simulink model "EvBoltCalib_Lat_v1_comb_GBSRoto"  (R2022b)
settings: configuration reference "ConfigSetDesktopFixedStep" (kept outside this file)
PreLoadFcn:
  | VSS_BICYCLE=Simulink.Variant('Dual=0');
  | VSS_DUAL=Simulink.Variant('Dual=1');
  | Dual=1;
model workspace (MAT data in the model file):
  Gas = 0.383333333333
undefined symbols (not defined in the file or in its folder): AccelCmd, ActTqLF_Nm_, ActTqLR_Nm_, ActTqRF_Nm_, ActTqRR_Nm_, BattChargeLimitMaxPwr, BattChargeLimitSocBpts, BattChargeLimitTbl, BattChrgCapcty, BattDischargeLimitSocBpts, BattDischargeLimitTbl, BattDischargeMaxPwr, BattNumCellsParallel, BattNumCellsSeries, BattOpenVoltCapBpts, BattOpenVoltTbl, BattResistSocBpts, BattResistTbl, BattResistTempBpts, BrakeMaxPrs, BrakeMaxTrq, ChassisDistCg2FrontAxle, ChassisDistCg2RearAxle, ChassisVehMass, CltchCmd, DecelCmd, DiffRatio, DiscIntNeverNeededParam, EnvGravCnst, EnvPrs, EnvTemp, FuelSpecificGrav, GearCmd, h, InitStates, lgSw, MtrEffSpdBpts, MtrEffTbl, MtrEffTrqBpts, MtrPwrMax, MtrTrqMax, SteeringCmd, SupvsryCtrlRegenBrkCutOffTbl, SupvsryCtrlRegenSpdBpts, TestScnrioCycleNum, VEH
libraries: VSIGenLib x39, simulink x25, etargetslib x24, vehdynlibtire x8, vehdynlibsuspension x7, vehdynlibtirecommon x7, autolibutils x5, autolibshared x5, CarMaker4SL x4, VsrLibWheel x4, sharedtransform x3, slrealtimeiplib x3
(part 11 of 11)

== system EvBoltCalib_Lat_v1_comb_GBSRoto/Subsystem/Vehicle/Vehicle Dynamics/Vehicle 14DOF/Wheels and Tires/VDBS/Tires/MF Tires/kappa ==
  In1 : Inport
  In2 : Inport  Port=2
  In3 : Inport  Port=3
  In4 : Inport  Port=4
  Bus Selector{,1..3} (4 alike) : BusSelector  OutputSignals=Kappa
  Vector Concatenate : Concatenate  NumInputs=4
  Out1 : Outport  VectorParamsAs1DForOutWhenUnconnected=off
  wires:
  Bus Selector3/1 -> Vector Concatenate/4  "<Kappa>"
  Bus Selector2/1 -> Vector Concatenate/3  "<Kappa>"
  Bus Selector1/1 -> Vector Concatenate/2  "<Kappa>"
  In4/1 -> Bus Selector3/1
  In3/1 -> Bus Selector2/1
  In2/1 -> Bus Selector1/1
  Bus Selector/1 -> Vector Concatenate/1  "<Kappa>"
  In1/1 -> Bus Selector/1
  Vector Concatenate/1 -> Out1/1

== system EvBoltCalib_Lat_v1_comb_GBSRoto/Subsystem/Vehicle/Vehicle Dynamics/Vehicle 14DOF/Wheels and Tires/VDBS/Tires/MF Tires/omega ==
  In1 : Inport
  In2 : Inport  Port=2
  In3 : Inport  Port=3
  In4 : Inport  Port=4
  Bus Selector{,1..3} (4 alike) : BusSelector  OutputSignals=Omega
  Vector Concatenate : Concatenate  NumInputs=4
  Out1 : Outport  VectorParamsAs1DForOutWhenUnconnected=off
  wires:
  In1/1 -> Bus Selector/1
  Bus Selector/1 -> Vector Concatenate/1  "<Omega>"
  In2/1 -> Bus Selector1/1
  In3/1 -> Bus Selector2/1
  In4/1 -> Bus Selector3/1
  Bus Selector1/1 -> Vector Concatenate/2  "<Omega>"
  Bus Selector2/1 -> Vector Concatenate/3  "<Omega>"
  Bus Selector3/1 -> Vector Concatenate/4  "<Omega>"
  Vector Concatenate/1 -> Out1/1

== system EvBoltCalib_Lat_v1_comb_GBSRoto/Subsystem/Vehicle/Vehicle Dynamics/Vehicle 14DOF/Wheels and Tires/VDBS/Tires/MF Tires/z ==
  In1 : Inport
  In2 : Inport  Port=2
  In3 : Inport  Port=3
  In4 : Inport  Port=4
  Bus Selector{,1..3} (4 alike) : BusSelector  OutputSignals=z
  Vector Concatenate : Concatenate  NumInputs=4
  Out1 : Outport  VectorParamsAs1DForOutWhenUnconnected=off
  wires:
  Bus Selector3/1 -> Vector Concatenate/4  "<z>"
  Bus Selector2/1 -> Vector Concatenate/3  "<z>"
  Bus Selector1/1 -> Vector Concatenate/2  "<z>"
  In4/1 -> Bus Selector3/1
  In3/1 -> Bus Selector2/1
  In2/1 -> Bus Selector1/1
  Bus Selector/1 -> Vector Concatenate/1  "<z>"
  In1/1 -> Bus Selector/1
  Vector Concatenate/1 -> Out1/1

== system EvBoltCalib_Lat_v1_comb_GBSRoto/Subsystem/Vehicle/Vehicle Dynamics/Vehicle 14DOF/Wheels and Tires/VDBS/Tires/MF Tires/zdot ==
  In1 : Inport
  In2 : Inport  Port=2
  In3 : Inport  Port=3
  In4 : Inport  Port=4
  Bus Selector{,1..3} (4 alike) : BusSelector  OutputSignals=zdot
  Vector Concatenate : Concatenate  NumInputs=4
  Out1 : Outport  VectorParamsAs1DForOutWhenUnconnected=off
  wires:
  Vector Concatenate/1 -> Out1/1
  In1/1 -> Bus Selector/1
  Bus Selector/1 -> Vector Concatenate/1  "<zdot>"
  In2/1 -> Bus Selector1/1
  In3/1 -> Bus Selector2/1
  In4/1 -> Bus Selector3/1
  Bus Selector1/1 -> Vector Concatenate/2  "<zdot>"
  Bus Selector2/1 -> Vector Concatenate/3  "<zdot>"
  Bus Selector3/1 -> Vector Concatenate/4  "<zdot>"

== matlab function EvBoltCalib_Lat_v1_comb_GBSRoto/Subsystem/Vehicle/Vehicle Dynamics/Vehicle 14DOF/Rototest and ORNL Interface/To Rototest with Band-Aid/RotoTestEthTx/MATLAB Function ==
  data: SpTqRR input; y output; SpTqLR input; SpTqRF input; SpTqLF input; SystemActive input
function y = fcn(SpTqRR, SpTqLR, SpTqRF, SpTqLF, SystemActive)

y = 0;
if SpTqRR == 1 && SystemActive == 0
    y = 30;
elseif SpTqRR == 0 && SystemActive == 0
    y = 0;
elseif SpTqRR == 1 && SystemActive == 1
    y = 31;
elseif SpTqRR == 0 && SystemActive == 1
    y = 1;
end

y = uint8(y);

== matlab function EvBoltCalib_Lat_v1_comb_GBSRoto/Subsystem/Vehicle/Vehicle Dynamics/Vehicle 7DOF/For 3D Visualization ==
  data: angles output size=3; angleIn input size=3; GeomXYZ output size=3; GemoXYZIn input size=3; GroundZ input size=4; trackW parameter; wheelB parameter
function [angles,GeomXYZ]= three26(angleIn, GemoXYZIn, GroundZ,trackW, wheelB)%#codegen
coder.allowpcode('plain')
% Copyright 2018 The MathWorks, Inc.
[angles,GeomXYZ]= vdynthree2six(angleIn, GemoXYZIn, GroundZ,trackW, wheelB);

== matlab function EvBoltCalib_Lat_v1_comb_GBSRoto/Subsystem/Vehicle/Vehicle Dynamics/Vehicle 14DOF/Rototest and ORNL Interface/Get Wheel Spd Cmd Based on Wheel Dynamics/Whl Dynamics & Format CM Powertrain Signal/Subsystem/MATLAB Function ==
  data: axleTorq input; switchFlag output; wheelSpd input
function switchFlag = fcn(axleTorq, wheelSpd)

% if braking and vehicle has stopped
if (abs(axleTorq) < 1e-5 && abs(wheelSpd) < 1e-5)
    switchFlag = 1;
else
    switchFlag = 0;
end

== matlab function EvBoltCalib_Lat_v1_comb_GBSRoto/Subsystem/Vehicle/Vehicle Dynamics/Vehicle 14DOF/Rototest and ORNL Interface/Get Wheel Spd Cmd Based on Wheel Dynamics/Whl Dynamics & Format CM Powertrain Signal/Subsystem2/MATLAB Function ==
  data: axleTorq input; switchFlag output; wheelSpd input
function switchFlag = fcn(axleTorq, wheelSpd)

% if braking and vehicle has stopped
if (abs(axleTorq) < 1e-5 && abs(wheelSpd) < 1e-5)
    switchFlag = 1;
else
    switchFlag = 0;
end

== matlab function EvBoltCalib_Lat_v1_comb_GBSRoto/Subsystem/Vehicle/Vehicle Dynamics/Vehicle 14DOF/Rototest and ORNL Interface/Get Wheel Spd Cmd Based on Wheel Dynamics/Whl Dynamics & Format CM Powertrain Signal/Subsystem3/MATLAB Function ==
  data: axleTorq input; switchFlag output; wheelSpd input
function switchFlag = fcn(axleTorq, wheelSpd)

% if braking and vehicle has stopped
if (abs(axleTorq) < 1e-5 && abs(wheelSpd) < 1e-5)
    switchFlag = 1;
else
    switchFlag = 0;
end

== matlab function EvBoltCalib_Lat_v1_comb_GBSRoto/Subsystem/Vehicle/Vehicle Dynamics/Vehicle 14DOF/Rototest and ORNL Interface/Get Wheel Spd Cmd Based on Wheel Dynamics/Whl Dynamics & Format CM Powertrain Signal/Subsystem4/MATLAB Function ==
  data: axleTorq input; switchFlag output; wheelSpd input
function switchFlag = fcn(axleTorq, wheelSpd)

% if braking and vehicle has stopped
if (abs(axleTorq) < 1e-5 && abs(wheelSpd) < 1e-5)
    switchFlag = 1;
else
    switchFlag = 0;
end

== stateflow chart EvBoltCalib_Lat_v1_comb_GBSRoto/Subsystem/Vehicle/Vehicle Dynamics/Vehicle 14DOF/Rototest and ORNL Interface/To Rototest with Band-Aid/Band-Aid/Band-Aid ==
  state dStop
    en:
    OutMode = 0;
    State = 3;
  state Running
    state SpeedMode
      en:
      OutMode = 1;
      state Blend
        en:
        OutSpd = InSpd;
        State = 0.1;
      state Driving
        du:
        OutSpd = InSpd;
        State = 0.2;
      (default) -> Blend
      Blend -> Driving
    state TorqueMode
      en:
      OutMode = 0;
      du:
      State = 1;
    (default) -> SpeedMode
    TorqueMode -> Blend : [after(SettleTime, sec) || ...
        | ~BrkSw]
    SpeedMode -> TorqueMode : [(any(InSpd < SpdLatchThr) && ...
        | (VehSpd_kph < VehSpdThr_kph) && BrkSw)]
  note: The vehicle will enter speed mode (driving) if:
      | The vehicle has been in torque mode for a calibrated time (settleTime) AND
      | The Input Speed (InSpd) is greater than a Launch Treshold (LaunchSpdThr) OR
      | The Input Torque (InTrq) is greater than calibrated torque value (LaunchTrqThr).
      | Criteria 1) sees the dyno has "settled" and allows the dyno to go back into speed mode.
      | Criteria 2) sees the vehicle is attempting to reaccelerate and pushes into speed mode.
      |
      | The vehicle will enter torque mode (zero) if:
      | Input Speed (InSpd) goes below the calibrated speed (SpdLatchThr) AND
      | Brake (BrkSw) is active.
      | 2) dStop is activated.
      | Criteria 1) sees the vehicle is attempting to come to a stop and unloads the dyno.
      | Criteria 2) is SHTF.
      |
      | && ...
      | (InSpd > LaunchSpdThr || ...
      | InTrq > LaunchTrqThr)
  (default) -> dStop
  Running -> dStop : [dStop]
  dStop -> Running : [~dStop]
  data: LaunchSpdThr input; LaunchTrqThr input; SpdLatchThr input; BrkSw input; InSpd input; InTrq input; OutMode output size=1; OutSpd output; State output; SettleTime input; dStop input; VehSpd_kph input; VehSpdThr_kph input
